simulink model "Temperature_Control_1"  (R2015b)
settings: Solver=VariableStepAuto  StartTime=0.0  StopTime=120  RelTol=1e-3
libraries: simulink x5
settings Model: Creator=vinayak  LastModifiedBy=vinayak

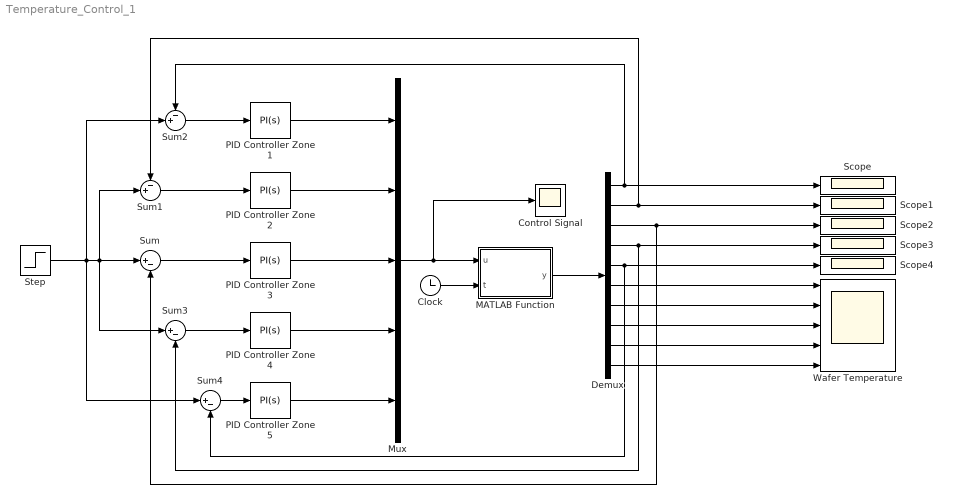
== system Temperature_Control_1 ==
  Clock : Clock
  Control Signal : Scope
  Demux : Demux  Outputs=10
  MATLAB Function : MATLAB Function  TreatAsAtomicUnit=on
  Mux : Mux  Inputs=5
  PID Controller Zone {1..3,5} (4 alike) : simulink/Continuous/PID Controller  Controller=PI  TimeDomain=Continuous-time  SampleTime=-1  IntegratorMethod=Forward Euler  FilterMethod=Forward Euler  Form=Parallel  UseFilter=on  ControllerParametersSource=internal  P=300  I=1  D=0  N=100  InitialConditionSource=internal  InitialConditionForIntegrator=0  InitialConditionForFilter=0  ExternalReset=none  LimitOutput=off  UpperSaturationLimit=inf  LowerSaturationLimit=-inf  LinearizeAsGain=on  AntiWindupMode=none  Kb=1  TrackingMode=off  Kt=1  PParamMin=[]  PParamMax=[]  IParamMin=[]  IParamMax=[]  DParamMin=[]  DParamMax=[]  NParamMin=[]  NParamMax=[]  KbParamMin=[]  KbParamMax=[]  KtParamMin=[]  KtParamMax=[]  POutMin=[]  POutMax=[]  IOutMin=[]  IOutMax=[]  DOutMin=[]  DOutMax=[]  NOutMin=[]  NOutMax=[]  KbOutMin=[]  KbOutMax=[]  KtOutMin=[]  KtOutMax=[]  IntegratorOutMin=[]  IntegratorOutMax=[]  FilterOutMin=[]  FilterOutMax=[]  SumOutMin=[]  SumOutMax=[]  SumI1OutMin=[]  SumI1OutMax=[]  SumI2OutMin=[]  SumI2OutMax=[]  SumI3OutMin=[]  SumI3OutMax=[]  SumDOutMin=[]  SumDOutMax=[]  SaturationOutMin=[]  SaturationOutMax=[]  IntegratorContinuousStateAttributes=''  IntegratorStateMustResolveToSignalObject=off  IntegratorRTWStateStorageClass=Auto  FilterContinuousStateAttributes=''  FilterStateMustResolveToSignalObject=off  FilterRTWStateStorageClass=Auto  DifferentiatorICPrevScaledInput=0  DifferentiatorOutMin=[]  DifferentiatorOutMax=[]
  "PID Controller Zone 4 " : simulink/Continuous/PID Controller  Controller=PI  TimeDomain=Continuous-time  SampleTime=-1  IntegratorMethod=Forward Euler  FilterMethod=Forward Euler  Form=Parallel  UseFilter=on  ControllerParametersSource=internal  P=300  I=1  D=0  N=100  InitialConditionSource=internal  InitialConditionForIntegrator=0  InitialConditionForFilter=0  ExternalReset=none  LimitOutput=off  UpperSaturationLimit=inf  LowerSaturationLimit=-inf  LinearizeAsGain=on  AntiWindupMode=none  Kb=1  TrackingMode=off  Kt=1  PParamMin=[]  PParamMax=[]  IParamMin=[]  IParamMax=[]  DParamMin=[]  DParamMax=[]  NParamMin=[]  NParamMax=[]  KbParamMin=[]  KbParamMax=[]  KtParamMin=[]  KtParamMax=[]  POutMin=[]  POutMax=[]  IOutMin=[]  IOutMax=[]  DOutMin=[]  DOutMax=[]  NOutMin=[]  NOutMax=[]  KbOutMin=[]  KbOutMax=[]  KtOutMin=[]  KtOutMax=[]  IntegratorOutMin=[]  IntegratorOutMax=[]  FilterOutMin=[]  FilterOutMax=[]  SumOutMin=[]  SumOutMax=[]  SumI1OutMin=[]  SumI1OutMax=[]  SumI2OutMin=[]  SumI2OutMax=[]  SumI3OutMin=[]  SumI3OutMax=[]  SumDOutMin=[]  SumDOutMax=[]  SaturationOutMin=[]  SaturationOutMax=[]  IntegratorContinuousStateAttributes=''  IntegratorStateMustResolveToSignalObject=off  IntegratorRTWStateStorageClass=Auto  FilterContinuousStateAttributes=''  FilterStateMustResolveToSignalObject=off  FilterRTWStateStorageClass=Auto  DifferentiatorICPrevScaledInput=0  DifferentiatorOutMin=[]  DifferentiatorOutMax=[]
  Scope{,1..4} (5 alike) : Scope
  Step : Step  Time=0  Before=90  After=90  SampleTime=0
  Sum : Sum  Inputs=|+-
  Sum1 : Sum  Inputs=-+|
  Sum2 : Sum  Inputs=-+|
  Sum3 : Sum  Inputs=|+-
  Sum4 : Sum  Inputs=|+-
  Wafer Temperature : Scope  NumInputPorts=5
  wires:
  Step/1 -> Sum4/1, Sum2/2, Sum3/1, Sum1/2, Sum/1
  Sum/1 -> PID Controller Zone 3/1
  Demux/2 -> Sum1/1, Scope1/1
  Demux/3 -> Scope2/1, Sum/2
  Demux/6 -> Wafer Temperature/1
  Demux/7 -> Wafer Temperature/2
  Demux/8 -> Wafer Temperature/3
  Demux/9 -> Wafer Temperature/4
  Demux/10 -> Wafer Temperature/5
  Demux/4 -> Scope3/1, Sum3/2
  Demux/5 -> Scope4/1, Sum4/2
  PID Controller Zone 3/1 -> Mux/3
  PID Controller Zone 1/1 -> Mux/1
  PID Controller Zone 2/1 -> Mux/2
  "PID Controller Zone 4 "/1 -> Mux/4
  PID Controller Zone 5/1 -> Mux/5
  Mux/1 -> MATLAB Function/1(u), Control Signal/1
  Sum1/1 -> PID Controller Zone 2/1
  Sum2/1 -> PID Controller Zone 1/1
  Sum4/1 -> PID Controller Zone 5/1
  Sum3/1 -> "PID Controller Zone 4 "/1
  Demux/1 -> Sum2/1, Scope/1
  MATLAB Function/1(y) -> Demux/1
  Clock/1 -> MATLAB Function/2(t)

== matlab function Temperature_Control_1/MATLAB Function ==
  data: u input; y output; t input
function y = fcn(u,t)
T1=[90 90 90 90 90 30 30 30 30 30];
T=T1';
Y=zeros(10,121)
Y(:,1)=T;
x=ibc_modelt(t,Y(:,t));
y = Y(:,t)+x;
Y(:,t+1)=y;
